simulink model "Middle_Ear_Filter"  (R2019b)
settings: Solver=VariableStepAuto  StartTime=0.0  StopTime=testtime  RelTol=1e-3
InitFcn:
  | Middle_Ear_Test_Parameters
StopFcn:
  | Verify_Middle_Ear
undefined symbols (not defined in the file or in its folder): dfilt, Fs, MEcoeffs, megainmax, MEscale
libraries: dsparch4 x2, dspsrcs4 x2
settings Model: Creator=mblun  LastModifiedBy=t96f346
settings OptimizationCC: BlockReduction=off  ConditionallyExecuteInputs=off  DefaultParameterBehavior=Inlined
settings DebuggingCC: AlgebraicLoopMsg=error
settings HardwareCC: ProdBitPerPointer=32  ProdBitPerSizeT=32  ProdBitPerPtrDiffT=32  ProdLargestAtomicFloat=None  ProdIntDivRoundTo=Undefined  ProdEndianess=Unspecified  ProdWordSize=32  ProdHWDeviceType=ASIC/FPGA->ASIC/FPGA  TargetBitPerPointer=64  TargetBitPerSizeT=64  TargetBitPerPtrDiffT=64  TargetLongLongMode=on  TargetIntDivRoundTo=Zero  TargetEndianess=LittleEndian  TargetWordSize=64  TargetHWDeviceType=Custom Processor->MATLAB Host Computer  ProdEqTarget=off
settings SFSimCC: CustomCodeUndefinedFunction=UseInterfaceOnly

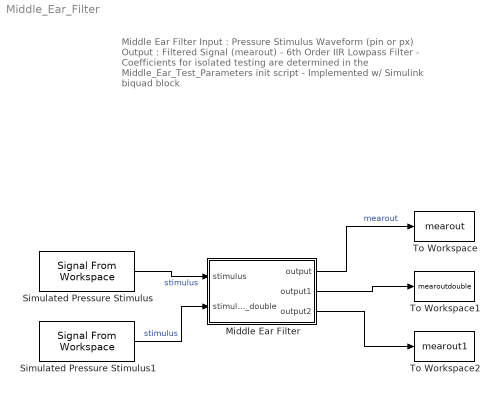
== system Middle_Ear_Filter ==
  note: Middle Ear Filter
      |
      | Input : Pressure Stimulus Waveform (pin or px)
      |
      | Output : Filtered Signal (mearout)
      |
      | - 6th Order IIR Lowpass Filter
      |
      | - Coefficients for isolated testing are determined in the Middle_Ear_Test_Parameters init script
      |
      | - Implemented w/ Simulink biquad block
  Middle Ear Filter : Subsystem
  Simulated Pressure Stimulus : dspsrcs4/Signal From Workspace  X=RxSignal  Ts=1/Fs  nsamps=1  OutputAfterFinalValue=Setting to zero  ignoreOrWarnInputAndFrameLengths=off  OutputFrames=off
  Simulated Pressure Stimulus1 : dspsrcs4/Signal From Workspace  X=RxSignalDouble  Ts=1/Fs  nsamps=1  OutputAfterFinalValue=Setting to zero  ignoreOrWarnInputAndFrameLengths=off  OutputFrames=off
  To Workspace : ToWorkspace  VariableName=mearout  SampleTime=-1
      settings: Save2DSignal=2-D array (concatenate along first dimension)
  To Workspace1 : ToWorkspace  VariableName=mearoutdouble  SampleTime=-1
      settings: Save2DSignal=2-D array (concatenate along first dimension)
  To Workspace2 : ToWorkspace  VariableName=mearout1  SampleTime=-1
      settings: Save2DSignal=2-D array (concatenate along first dimension)
  wires:
  Simulated Pressure Stimulus/1 -> Middle Ear Filter/1(stimulus)  "stimulus"
  Middle Ear Filter/1(output) -> To Workspace/1  "mearout"
  Simulated Pressure Stimulus1/1 -> Middle Ear Filter/2(stimulus_double)  "stimulus"
  Middle Ear Filter/2(output1) -> To Workspace1/1
  Middle Ear Filter/3(output2) -> To Workspace2/1

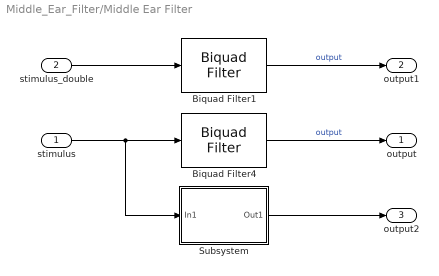
== system Middle_Ear_Filter/Middle Ear Filter ==
  stimulus : Inport
  stimulus_double : Inport  Port=2
  Biquad Filter1 : dsparch4/Biquad Filter  FilterSource=Dialog parameters  CoeffSource=Specify via dialog  FilterObject=dfilt.df2tsos([1 0.3 0.4],[1 0.1 0.2])  IIRFiltStruct=Direct form I  BiQuadCoeffs=MEcoeffs  ScaleValues=[1 1 1 1/megainmax]  IC=0  ICnum=0  ICden=0  a0Flag=Warning  optimizeScaleValues=on  ScaleValueMode=Specify via input port (g)  roundingMode=Floor  overflowMode=on  scaleValueFracLength=14  denProdOutputFracLength=30  denAccumFracLength=30  secondMemoryFracLength=15
      settings: SourceProductName=DSP System Toolbox
  Biquad Filter4 : dsparch4/Biquad Filter  FilterSource=Dialog parameters  CoeffSource=Specify via dialog  FilterObject=dfilt.df2tsos([1 0.3 0.4],[1 0.1 0.2])  IIRFiltStruct=Direct form I  BiQuadCoeffs=MEcoeffs  ScaleValues=[1 1 1 MEscale]  IC=0  ICnum=0  ICden=0  a0Flag=Warning  optimizeScaleValues=on  ScaleValueMode=Specify via input port (g)  roundingMode=Floor  overflowMode=on  scaleValueFracLength=14  denProdOutputFracLength=30  denAccumFracLength=30  secondMemoryFracLength=15
      settings: SourceProductName=DSP System Toolbox
  Subsystem : Subsystem
  output : Outport  VectorParamsAs1DForOutWhenUnconnected=off
  output1 : Outport  Port=2  VectorParamsAs1DForOutWhenUnconnected=off
  output2 : Outport  Port=3  VectorParamsAs1DForOutWhenUnconnected=off
  wires:
  stimulus/1 -> Subsystem/1(In1), Biquad Filter4/1
  Biquad Filter4/1 -> output/1  "output"
  Biquad Filter1/1 -> output1/1  "output"
  stimulus_double/1 -> Biquad Filter1/1
  Subsystem/1(Out1) -> output2/1

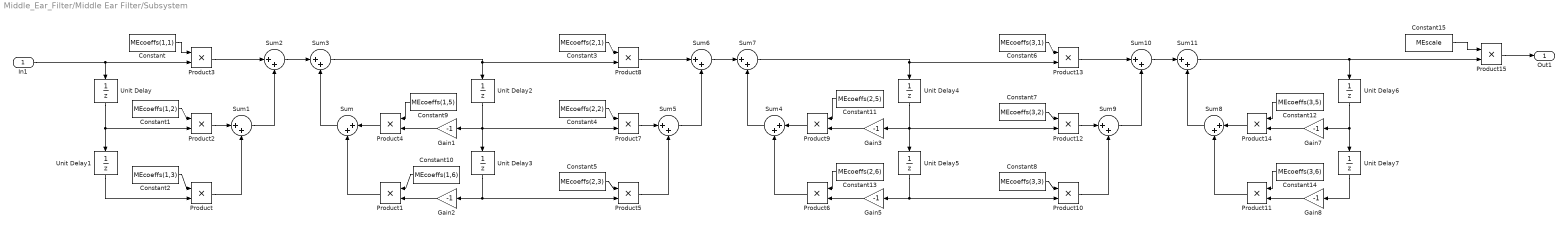
== system Middle_Ear_Filter/Middle Ear Filter/Subsystem ==
  In1 : Inport
  Constant : Constant  Value=MEcoeffs(1,1)  OutDataTypeStr=single  SampleTime=-1
  Constant1 : Constant  Value=MEcoeffs(1,2)  OutDataTypeStr=single  SampleTime=-1
  Constant10 : Constant  Value=MEcoeffs(1,6)  OutDataTypeStr=single  SampleTime=-1
  Constant11 : Constant  Value=MEcoeffs(2,5)  OutDataTypeStr=single  SampleTime=-1
  Constant12 : Constant  Value=MEcoeffs(3,5)  OutDataTypeStr=single  SampleTime=-1
  Constant13 : Constant  Value=MEcoeffs(2,6)  OutDataTypeStr=single  SampleTime=-1
  Constant14 : Constant  Value=MEcoeffs(3,6)  OutDataTypeStr=single  SampleTime=-1
  Constant15 : Constant  Value=MEscale  OutDataTypeStr=single  SampleTime=-1
  Constant2 : Constant  Value=MEcoeffs(1,3)  OutDataTypeStr=single  SampleTime=-1
  Constant3 : Constant  Value=MEcoeffs(2,1)  OutDataTypeStr=single  SampleTime=-1
  Constant4 : Constant  Value=MEcoeffs(2,2)  OutDataTypeStr=single  SampleTime=-1
  Constant5 : Constant  Value=MEcoeffs(2,3)  OutDataTypeStr=single  SampleTime=-1
  Constant6 : Constant  Value=MEcoeffs(3,1)  OutDataTypeStr=single  SampleTime=-1
  Constant7 : Constant  Value=MEcoeffs(3,2)  OutDataTypeStr=single  SampleTime=-1
  Constant8 : Constant  Value=MEcoeffs(3,3)  OutDataTypeStr=single  SampleTime=-1
  Constant9 : Constant  Value=MEcoeffs(1,5)  OutDataTypeStr=single  SampleTime=-1
  Gain{1..3,5,7..8} (6 alike) : Gain  Gain=-1
  Product{,1..15} (16 alike) : Product
  Sum{,1..11} (12 alike) : Sum  Inputs=|++
  Unit Delay{,1..7} (8 alike) : UnitDelay  SampleTime=-1  HasFrameUpgradeWarning=on
  Out1 : Outport
  wires:
  Product/1 -> Sum1/2
  Gain5/1 -> Product6/2
  Constant9/1 -> Product4/1
  Gain8/1 -> Product11/2
  Unit Delay1/1 -> Product/2
  Sum6/1 -> Sum7/1
  Gain2/1 -> Product1/2
  Product8/1 -> Sum6/1
  Gain3/1 -> Product9/2
  Sum10/1 -> Sum11/1
  Product9/1 -> Sum4/1
  Unit Delay6/1 -> Unit Delay7/1, Gain7/1
  Unit Delay3/1 -> Product5/2, Gain2/1
  Product6/1 -> Sum4/2
  Unit Delay5/1 -> Product10/2, Gain5/1
  Product13/1 -> Sum10/1
  Product5/1 -> Sum5/2
  Unit Delay7/1 -> Gain8/1
  Product2/1 -> Sum1/1
  Product14/1 -> Sum8/1
  Product10/1 -> Sum9/2
  Sum2/1 -> Sum3/1
  Sum11/1 -> Product15/2, Unit Delay6/1
  Unit Delay4/1 -> Product12/2, Unit Delay5/1, Gain3/1
  Product3/1 -> Sum2/1
  Sum/1 -> Sum3/2
  Sum3/1 -> Product8/2, Unit Delay2/1
  Product12/1 -> Sum9/1
  Sum8/1 -> Sum11/2
  Sum7/1 -> Product13/2, Unit Delay4/1
  Product7/1 -> Sum5/1
  Sum4/1 -> Sum7/2
  Sum5/1 -> Sum6/2
  In1/1 -> Product3/2, Unit Delay/1
  Sum9/1 -> Sum10/2
  Unit Delay2/1 -> Product7/2, Unit Delay3/1, Gain1/1
  Constant/1 -> Product3/1
  Product1/1 -> Sum/2
  Sum1/1 -> Sum2/2
  Product11/1 -> Sum8/2
  Gain1/1 -> Product4/2
  Product4/1 -> Sum/1
  Gain7/1 -> Product14/2
  Unit Delay/1 -> Unit Delay1/1, Product2/2
  Constant1/1 -> Product2/1
  Constant3/1 -> Product8/1
  Constant4/1 -> Product7/1
  Constant5/1 -> Product5/1
  Constant6/1 -> Product13/1
  Constant7/1 -> Product12/1
  Constant8/1 -> Product10/1
  Constant2/1 -> Product/1
  Constant10/1 -> Product1/1
  Constant11/1 -> Product9/1
  Constant13/1 -> Product6/1
  Constant14/1 -> Product11/1
  Constant12/1 -> Product14/1
  Constant15/1 -> Product15/1
  Product15/1 -> Out1/1
